simulink model "estimacao_Ktau"  (R2020b)
settings: Solver=VariableStepAuto  StartTime=0.0  StopTime=10  RelTol=1e-3
values from neighbouring files (symbols this model uses):
  A = A    [minquad.m]    (also in motor.mat = [-676.470588235  -206.018789225; 26.2510368664  -1.405913978)
  B = [294.117647059 0]    [motor.mat]
  C = [0 1]    [motor.mat]
  K_area = 1.2    [K_tau_estimados.mat]
  K_bode = 1.1768    [K_tau_estimados.mat]
  K_fun = 1.2    [K_tau_estimados.mat]
  K_nep = 1.2    [K_tau_estimados.mat]    (also in exp4.m = 1.2, K_fun = K_nep, K_area = K_fun)
  Kt = 0.0215571428571    [motor.mat]
  tau_area = 0.1077    [K_tau_estimados.mat]    (also in exp4.m = tau_area(steptime,initialvalue,finalvalue,times,values))
  tau_bode = 0.1279    [K_tau_estimados.mat]
  tau_fun = 0.086    [K_tau_estimados.mat]    (also in exp4.m = tau_funcao(steptime,initialvalue,finalvalue,times,values))
  tau_nep = 0.1091    [K_tau_estimados.mat]    (also in exp4.m = tau_nep(steptime,initialvalue,finalvalue,times,values))
libraries: simulink x8
settings Model: Creator=gusta  LastModifiedBy=lucas
settings DebuggingCC: SFMachineParentedDataDiag=error

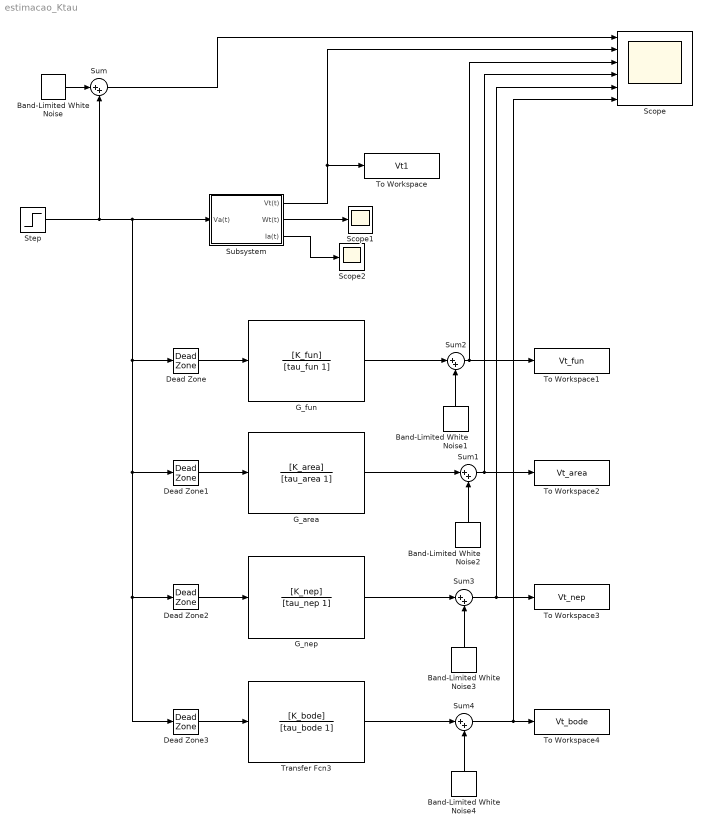
== system estimacao_Ktau ==
  Band-Limited White Noise : simulink/Sources/Band-Limited White Noise  Cov=[0.000001]  Ts=0.001  seed=[23341]
  Band-Limited White Noise{1..4} (4 alike) : simulink/Sources/Band-Limited White Noise  Cov=[0.00000001]  Ts=0.001  seed=[23341]
  Dead Zone{,1..3} (4 alike) : DeadZone  LowerValue=-3.2  UpperValue=3.2  SaturateOnIntegerOverflow=on
  G_area : TransferFcn  Numerator=[K_area]  Denominator=[tau_area 1]
  G_fun : TransferFcn  Numerator=[K_fun]  Denominator=[tau_fun 1]
  G_nep : TransferFcn  Numerator=[K_nep]  Denominator=[tau_nep 1]
  Scope : Scope  NumInputPorts=6
  Scope1 : Scope
  Scope2 : Scope
  Step : Step  Time=0  After=10  SampleTime=0
  Subsystem : Subsystem
  Sum{,1..4} (5 alike) : Sum  Inputs=|++
  To Workspace : ToWorkspace  VariableName=Vt1  SaveFormat=Structure With Time  SampleTime=-1
  To Workspace1 : ToWorkspace  VariableName=Vt_fun  SaveFormat=Structure With Time  SampleTime=-1
  To Workspace2 : ToWorkspace  VariableName=Vt_area  SaveFormat=Structure With Time  SampleTime=-1
  To Workspace3 : ToWorkspace  VariableName=Vt_nep  SaveFormat=Structure With Time  SampleTime=-1
  To Workspace4 : ToWorkspace  VariableName=Vt_bode  SaveFormat=Structure With Time  SampleTime=-1
  Transfer Fcn3 : TransferFcn  Numerator=[K_bode]  Denominator=[tau_bode 1]
  wires:
  Subsystem/1(Vt(t)) -> To Workspace/1, Scope/2
  Subsystem/2(Wt(t)) -> Scope1/1
  Subsystem/3(Ia(t)) -> Scope2/1
  Step/1 -> Sum/2, Subsystem/1(Va(t)), Dead Zone/1, Dead Zone3/1, Dead Zone2/1, Dead Zone1/1
  G_fun/1 -> Sum2/1
  G_area/1 -> Sum1/1
  G_nep/1 -> Sum3/1
  Transfer Fcn3/1 -> Sum4/1
  Dead Zone/1 -> G_fun/1
  Dead Zone1/1 -> G_area/1
  Dead Zone2/1 -> G_nep/1
  Dead Zone3/1 -> Transfer Fcn3/1
  Band-Limited White Noise/1 -> Sum/1
  Sum/1 -> Scope/1
  Band-Limited White Noise1/1 -> Sum2/2
  Sum2/1 -> To Workspace1/1, Scope/3
  Band-Limited White Noise2/1 -> Sum1/2
  Sum1/1 -> To Workspace2/1, Scope/4
  Band-Limited White Noise3/1 -> Sum3/2
  Sum3/1 -> Scope/5, To Workspace3/1
  Band-Limited White Noise4/1 -> Sum4/2
  Sum4/1 -> To Workspace4/1, Scope/6

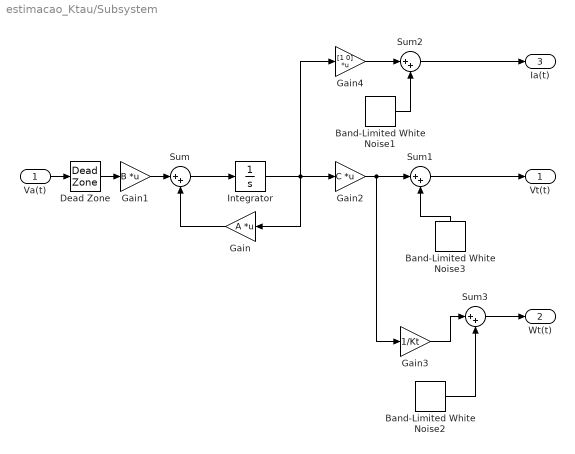
== system estimacao_Ktau/Subsystem ==
  Va(t) : Inport
  Band-Limited White Noise1 : simulink/Sources/Band-Limited White Noise  Cov=[0.00000001]  Ts=0.001  seed=[23341]
  Band-Limited White Noise2 : simulink/Sources/Band-Limited White Noise  Cov=[0.0007]  Ts=0.001  seed=[23341]
  Band-Limited White Noise3 : simulink/Sources/Band-Limited White Noise  Cov=[0.00000001]  Ts=0.001  seed=[23341]
  Dead Zone : DeadZone  LowerValue=-3.2  UpperValue=3.2  SaturateOnIntegerOverflow=on
  Gain : Gain  Gain=A  Multiplication=Matrix(K*u)
  Gain1 : Gain  Gain=B  Multiplication=Matrix(K*u)
  Gain2 : Gain  Gain=C  Multiplication=Matrix(K*u)
  Gain3 : Gain  Gain=1/Kt
  Gain4 : Gain  Gain=[1 0]  Multiplication=Matrix(K*u)
  Integrator : Integrator
  Sum{,1..3} (4 alike) : Sum  Inputs=|++
  Vt(t) : Outport
  Wt(t) : Outport  Port=2
  Ia(t) : Outport  Port=3
  wires:
  Sum/1 -> Integrator/1
  Integrator/1 -> Gain4/1, Gain2/1, Gain/1
  Gain1/1 -> Sum/1
  Gain/1 -> Sum/2
  Va(t)/1 -> Dead Zone/1
  Dead Zone/1 -> Gain1/1
  Sum2/1 -> Ia(t)/1
  Gain4/1 -> Sum2/1
  Sum3/1 -> Wt(t)/1
  Band-Limited White Noise1/1 -> Sum2/2
  Band-Limited White Noise2/1 -> Sum3/2
  Gain3/1 -> Sum3/1
  Gain2/1 -> Sum1/1, Gain3/1
  Band-Limited White Noise3/1 -> Sum1/2
  Sum1/1 -> Vt(t)/1
